simulink model "cbf"  (R2021a)
settings: Solver=FixedStepAuto  StartTime=0.0  StopTime=inf  FixedStep=0.05  RelTol=1e-3
undefined symbols (not defined in the file): Angular, Linear
libraries: robotlib x34
settings Model: Creator=ivory  LastModifiedBy=sprinkle
settings SolverCC: AlgebraicLoopSolver=TrustRegion
settings OptimizationCC: EnhancedBackFolding=on  PassReuseOutputArgsAs=Individual arguments  ZeroExternalMemoryAtStartup=off  ZeroInternalMemoryAtStartup=off  MaxStackSize=64  OptimizeBlockOrder=speed  DifferentSizesBufferReuse=on  OptimizationCustomize=off  EfficientTunableParamExpr=on
settings DebuggingCC: ParameterTunabilityLossMsg=error  SFMachineParentedDataDiag=warning
settings HardwareCC: ProdBitPerPointer=32  ProdBitPerSizeT=32  ProdBitPerPtrDiffT=32  ProdLargestAtomicFloat=None  ProdIntDivRoundTo=Undefined  ProdEndianess=Unspecified  ProdWordSize=32  ProdHWDeviceType=Generic->Unspecified (assume 32-bit Generic)
settings SFSimCC: MATLABDynamicMemAlloc=off  SimTargetLang=C++
settings RTWCC: SystemTargetFile=ert.tlc  HardwareBoard=Robot Operating System (ROS)  TLCOptions="-aInlineSetEventsForThisBaseRateFcn=TLC_FALSE -aSuppressMultiTaskScheduler=TLC_FALSE  -aRateBasedStepFcn=0"  TemplateMakefile=ert_default_tmf  GenerateReport=on  Toolchain=Catkin  IncludeHyperlinkInReport=on  LaunchReport=on  TargetLang=C++  GenerateTraceInfo=on  GenerateTraceReport=on  GenerateTraceReportSl=on  GenerateTraceReportSf=on  GenerateTraceReportEml=on
settings CodeAppCC: ForceParamTrailComments=on  IgnoreCustomStorageClasses=off  OperatorAnnotations=on  SimulinkDataObjDesc=on  SFDataObjDesc=on  InsertBlockDesc=on
settings ERTTargetCC: SupportContinuousTime=on  SupportVariableSizeSignals=on

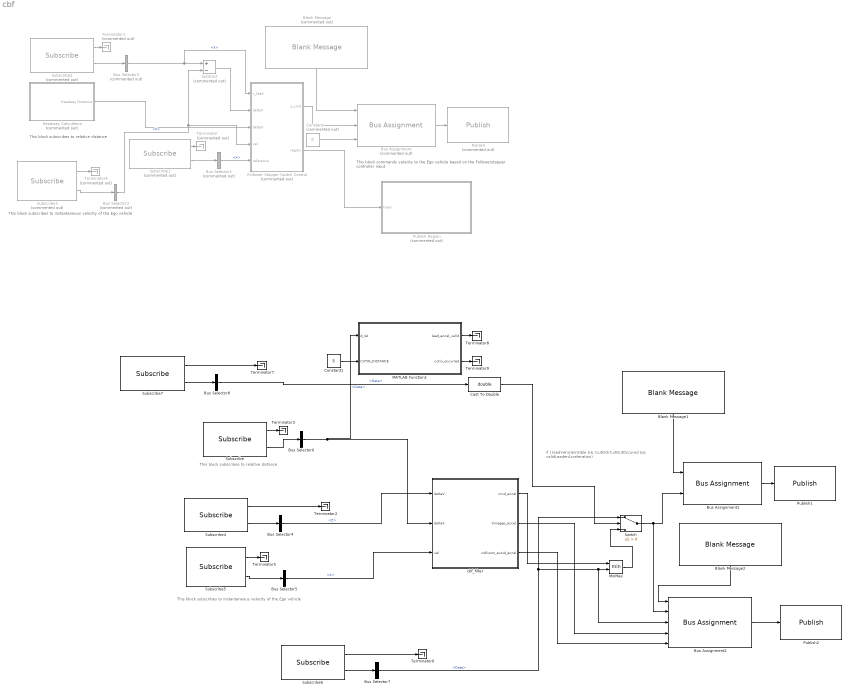
== system cbf ==
  note: if ( leadVehicleVisible && !cutInOrCutOutOccured && validLeaderAcceleration)
  note: This block subscribes to
      | instantaneous velocity of the Ego vehicle
  note: This block subscribes
      | to relative distance
  note: This block commands velocity to the Ego vehicle based
      | on the Followerstopper controller input
  note: This block subscribes
      | to relative distance
  note: This block subscribes to
      | instantaneous velocity of the Ego vehicle
  Blank Message : robotlib/Blank Message  Commented=on  messageClass=Message  entityType=geometry_msgs/Twist  messageType=geometry_msgs/Twist  SampleTime=inf  legacyBusStruct=off
  Blank Message1 : robotlib/Blank Message  messageClass=Message  entityType=std_msgs/Float64  messageType=std_msgs/Float64  SampleTime=inf  legacyBusStruct=off
  Blank Message2 : robotlib/Blank Message  messageClass=Message  entityType=geometry_msgs/Twist  messageType=geometry_msgs/Twist  SampleTime=inf  legacyBusStruct=off
  Bus Assignment : BusAssignment  Commented=on  AssignedSignals=Linear.X,Angular.Z
  Bus Assignment1 : BusAssignment  AssignedSignals=Data
  Bus Assignment2 : BusAssignment  AssignedSignals=Linear.X,Linear.Y,Angular.Y,Angular.Z
  Bus Selector1 : BusSelector  Commented=on  OutputSignals=Linear.X
  Bus Selector2 : BusSelector  Commented=on  OutputSignals=Linear.X
  Bus Selector3 : BusSelector  Commented=on  OutputSignals=Linear.X
  Bus Selector4 : BusSelector  OutputSignals=Linear.Z
  Bus Selector5 : BusSelector  OutputSignals=Linear.X
  Bus Selector6 : BusSelector  OutputSignals=Data
  Bus Selector7 : BusSelector  OutputSignals=Data
  Bus Selector8 : BusSelector  OutputSignals=Data
  Cast To Double : DataTypeConversion  OutDataTypeStr=double
  Constant : Constant  Commented=on  Value=0
  Constant1 : Constant  Value=5
  Follower Stopper Switch Control : Subsystem  Commented=on
  Headway Calculation : Subsystem  Commented=on
  MATLAB Function1 : MATLAB Function  TreatAsAtomicUnit=on
  MinMax : MinMax  Inputs=2
  Publish : robotlib/Publish  Commented=on  topicSource=Specify your own  topic=cmd_vel  messageType=geometry_msgs/Twist  legacyBusStruct=off  messageQueueLength=1
  Publish Region : Subsystem  Commented=on
  Publish1 : robotlib/Publish  topicSource=Specify your own  topic=cmd_accel  messageType=std_msgs/Float64  legacyBusStruct=off  messageQueueLength=1
  Publish2 : robotlib/Publish  topicSource=Specify your own  topic=/cbf/cbf_debug  messageType=geometry_msgs/Twist  legacyBusStruct=off  messageQueueLength=1
  Subscribe : robotlib/Subscribe  topicSource=Specify your own  topic=lead_dist  messageType=std_msgs/Float64  SampleTime=-1  legacyBusStruct=off  messageQueueLength=1
  Subscribe1 : robotlib/Subscribe  Commented=on  topicSource=Specify your own  topic=v_ref  messageType=geometry_msgs/Twist  SampleTime=-1  legacyBusStruct=off  messageQueueLength=1
  Subscribe2 : robotlib/Subscribe  Commented=on  topicSource=Specify your own  topic=leader_vel  messageType=geometry_msgs/Twist  SampleTime=-1  legacyBusStruct=off  messageQueueLength=1
  Subscribe3 : robotlib/Subscribe  Commented=on  topicSource=Specify your own  topic=vel  messageType=geometry_msgs/Twist  SampleTime=-1  legacyBusStruct=off  messageQueueLength=1
  Subscribe4 : robotlib/Subscribe  topicSource=Specify your own  topic=rel_vel  messageType=geometry_msgs/Twist  SampleTime=-1  legacyBusStruct=off  messageQueueLength=1
  Subscribe5 : robotlib/Subscribe  topicSource=Specify your own  topic=vel  messageType=geometry_msgs/Twist  SampleTime=-1  legacyBusStruct=off  messageQueueLength=1
  Subscribe6 : robotlib/Subscribe  topicSource=Specify your own  topic=cmd_accel_pre  messageType=std_msgs/Float64  SampleTime=-1  legacyBusStruct=off  messageQueueLength=1
  Subscribe7 : robotlib/Subscribe  topicSource=Specify your own  topic=/car/hud/mini_car_enable  messageType=std_msgs/Bool  SampleTime=-1  legacyBusStruct=off  messageQueueLength=1
  Subtract : Sum  Commented=on  Inputs=+-
  Switch : Switch  Criteria=u2 > Threshold
  Terminator : Terminator  Commented=on
  Terminator1 : Terminator  Commented=on
  Terminator{2..3,5..9} (7 alike) : Terminator
  Terminator4 : Terminator  Commented=on
  cbf_filter : Subsystem
  wires:
  Bus Assignment/1 -> Publish/1
  Subscribe3/2 -> Bus Selector3/1
  Blank Message/1 -> Bus Assignment/1
  Bus Selector3/1 -> Subtract/2, Follower Stopper Switch Control/4(vel)  "<X>"
  Constant/1 -> Bus Assignment/3
  Subscribe3/1 -> Terminator4/1
  Follower Stopper Switch Control/1(u_cmd) -> Bus Assignment/2
  Headway Calculation/1(Headway Distance) -> Follower Stopper Switch Control/3(deltaX)
  Bus Selector1/1 -> Follower Stopper Switch Control/5(reference)  "<X>"
  Follower Stopper Switch Control/2(region) -> Publish Region/1(Input)
  Subscribe1/1 -> Terminator/1
  Subscribe1/2 -> Bus Selector1/1
  Subscribe2/2 -> Bus Selector2/1
  Bus Selector2/1 -> Follower Stopper Switch Control/1(v_lead), Subtract/1  "<X>"
  Subtract/1 -> Follower Stopper Switch Control/2(deltaV)
  Subscribe2/1 -> Terminator1/1
  Subscribe4/1 -> Terminator2/1
  Bus Selector4/1 -> cbf_filter/1(deltaV)  "<Z>"
  Subscribe5/2 -> Bus Selector5/1
  Subscribe4/2 -> Bus Selector4/1
  Bus Selector5/1 -> cbf_filter/3(vel)  "<X>"
  Bus Assignment1/1 -> Publish1/1
  Blank Message1/1 -> Bus Assignment1/1
  Subscribe5/1 -> Terminator5/1
  Subscribe/1 -> Terminator3/1
  Subscribe/2 -> Bus Selector6/1
  Bus Selector6/1 -> MATLAB Function1/1(d_rel), cbf_filter/2(deltaX)  "<Data>"
  Subscribe6/2 -> Bus Selector7/1
  Bus Selector7/1 -> Switch/1, Bus Assignment2/3, MinMax/2  "<Data>"
  Subscribe6/1 -> Terminator6/1
  Subscribe7/2 -> Bus Selector8/1
  Subscribe7/1 -> Terminator7/1
  Bus Selector8/1 -> Cast To Double/1  "<Data>"
  Constant1/1 -> MATLAB Function1/2(CUTIN_DISTANCE)
  cbf_filter/1(cmd_accel) -> MinMax/1
  MinMax/1 -> Switch/3
  Switch/1 -> Bus Assignment2/2, Bus Assignment1/2
  Blank Message2/1 -> Bus Assignment2/1
  Bus Assignment2/1 -> Publish2/1
  cbf_filter/2(timegap_accel) -> Bus Assignment2/4
  cbf_filter/3(collision_avoid_accel) -> Bus Assignment2/5
  Cast To Double/1 -> Switch/2
  MATLAB Function1/1(lead_accel_valid) -> Terminator8/1
  MATLAB Function1/2(cutin_occurred) -> Terminator9/1

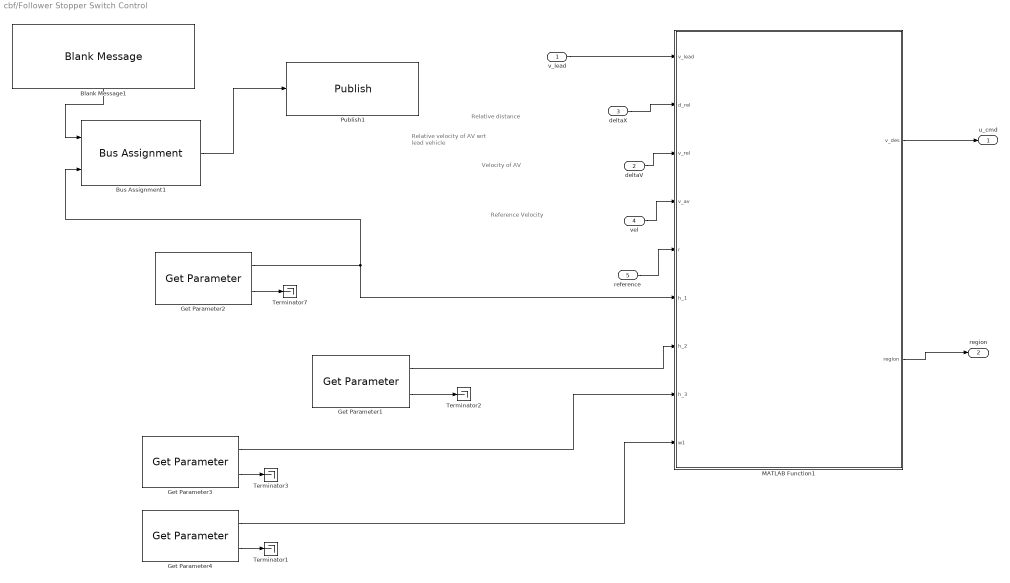
== system cbf/Follower Stopper Switch Control ==
  note: Relative velocity of
      | AV wrt lead vehicle
  note: Velocity of AV
  note: Reference Velocity
  note: Relative distance
  v_lead : Inport
  deltaV : Inport  Port=2
  deltaX : Inport  Port=3
  vel : Inport  Port=4
  reference : Inport  Port=5
  Blank Message1 : robotlib/Blank Message  messageClass=Message  entityType=std_msgs/Float64  messageType=std_msgs/Float64  SampleTime=inf  legacyBusStruct=off
  Bus Assignment1 : BusAssignment  AssignedSignals=Data
  Get Parameter1 : robotlib/Get Parameter  ParameterSource=Specify your own  ParameterName=th2  ParameterType=double  ParameterMaxArrayLength=16  ParameterInitialValue=1.2  SampleTime=-1  ShowErrorCodeOutput=on  ModelName=followerstoppermax  BlockId=ParamGet_followerstoppermax_228
      settings: SourceProductBaseCode=RR
  Get Parameter2 : robotlib/Get Parameter  ParameterSource=Specify your own  ParameterName=th1  ParameterType=double  ParameterMaxArrayLength=16  ParameterInitialValue=0.4  SampleTime=-1  ShowErrorCodeOutput=on  ModelName=followerstoppermax  BlockId=ParamGet_followerstoppermax_226
      settings: SourceProductBaseCode=RR
  Get Parameter3 : robotlib/Get Parameter  ParameterSource=Specify your own  ParameterName=th3  ParameterType=double  ParameterMaxArrayLength=16  ParameterInitialValue=1.8  SampleTime=-1  ShowErrorCodeOutput=on  ModelName=followerstoppermax  BlockId=ParamGet_followerstoppermax_230
      settings: SourceProductBaseCode=RR
  Get Parameter4 : robotlib/Get Parameter  ParameterSource=Specify your own  ParameterName=w1  ParameterType=double  ParameterMaxArrayLength=16  ParameterInitialValue=4.5  SampleTime=-1  ShowErrorCodeOutput=on  ModelName=followerstoppermax  BlockId=ParamGet_followerstoppermax_235
      settings: SourceProductBaseCode=RR
  MATLAB Function1 : MATLAB Function  TreatAsAtomicUnit=on
  Publish1 : robotlib/Publish  topicSource=Specify your own  topic=timheadway1  messageType=std_msgs/Float64  legacyBusStruct=off  messageQueueLength=1
  Terminator{1..3,7} (4 alike) : Terminator
  u_cmd : Outport
  region : Outport  Port=2
  wires:
  deltaX/1 -> MATLAB Function1/2(d_rel)
  deltaV/1 -> MATLAB Function1/3(v_rel)
  vel/1 -> MATLAB Function1/4(v_av)
  v_lead/1 -> MATLAB Function1/1(v_lead)
  reference/1 -> MATLAB Function1/5(r)
  MATLAB Function1/1(v_des) -> u_cmd/1
  MATLAB Function1/2(region) -> region/1
  Get Parameter3/1 -> MATLAB Function1/8(h_3)
  Get Parameter1/2 -> Terminator2/1
  Get Parameter1/1 -> MATLAB Function1/7(h_2)
  Get Parameter3/2 -> Terminator3/1
  Get Parameter2/2 -> Terminator7/1
  Blank Message1/1 -> Bus Assignment1/1
  Bus Assignment1/1 -> Publish1/1
  Get Parameter2/1 -> Bus Assignment1/2, MATLAB Function1/6(h_1)
  Get Parameter4/2 -> Terminator1/1
  Get Parameter4/1 -> MATLAB Function1/9(w1)

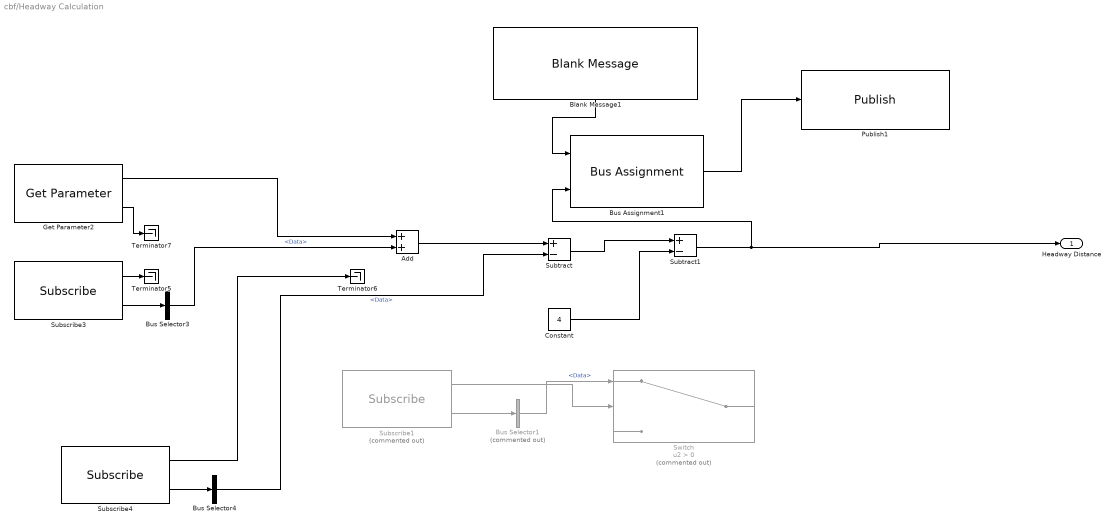
== system cbf/Headway Calculation ==
  Add : Sum
  Blank Message1 : robotlib/Blank Message  messageClass=Message  entityType=std_msgs/Float64  messageType=std_msgs/Float64  SampleTime=inf  legacyBusStruct=off
  Bus Assignment1 : BusAssignment  AssignedSignals=Data
  Bus Selector1 : BusSelector  Commented=on  OutputSignals=Data
  Bus Selector3 : BusSelector  OutputSignals=Data
  Bus Selector4 : BusSelector  OutputSignals=Data
  Constant : Constant  Value=4
  Get Parameter2 : robotlib/Get Parameter  ParameterSource=Specify your own  ParameterName=init_gap  ParameterType=double  ParameterMaxArrayLength=16  ParameterInitialValue=30.0  SampleTime=-1  ShowErrorCodeOutput=on  ModelName=fs_th  BlockId=ParamGet_fs_th_177
      settings: SourceProductBaseCode=RR
  Publish1 : robotlib/Publish  topicSource=Specify your own  topic=headway_est  messageType=std_msgs/Float64  legacyBusStruct=off  messageQueueLength=1
  Subscribe1 : robotlib/Subscribe  Commented=on  topicSource=Specify your own  topic=headway  messageType=std_msgs/Float64  SampleTime=-1  legacyBusStruct=off  messageQueueLength=1
  Subscribe3 : robotlib/Subscribe  topicSource=Specify your own  topic=leader_dist_x  messageType=std_msgs/Float64  SampleTime=-1  legacyBusStruct=off  messageQueueLength=1
  Subscribe4 : robotlib/Subscribe  topicSource=Specify your own  topic=dist_x  messageType=std_msgs/Float64  SampleTime=-1  legacyBusStruct=off  messageQueueLength=1
  Subtract : Sum  Inputs=+-
  Subtract1 : Sum  Inputs=+-
  Switch : Switch  Commented=on  Criteria=u2 > Threshold
  Terminator5 : Terminator
  Terminator6 : Terminator
  Terminator7 : Terminator
  Headway Distance : Outport
  wires:
  Bus Selector3/1 -> Add/2  "<Data>"
  Subscribe1/2 -> Bus Selector1/1
  Subscribe3/2 -> Bus Selector3/1
  Subscribe4/1 -> Terminator6/1
  Bus Selector1/1 -> Switch/1  "<Data>"
  Subscribe1/1 -> Switch/2
  Bus Selector4/1 -> Subtract/2  "<Data>"
  Get Parameter2/2 -> Terminator7/1
  Subscribe4/2 -> Bus Selector4/1
  Get Parameter2/1 -> Add/1
  Subscribe3/1 -> Terminator5/1
  Add/1 -> Subtract/1
  Subtract/1 -> Subtract1/1
  Blank Message1/1 -> Bus Assignment1/1
  Bus Assignment1/1 -> Publish1/1
  Subtract1/1 -> Bus Assignment1/2, Headway Distance/1
  Constant/1 -> Subtract1/2

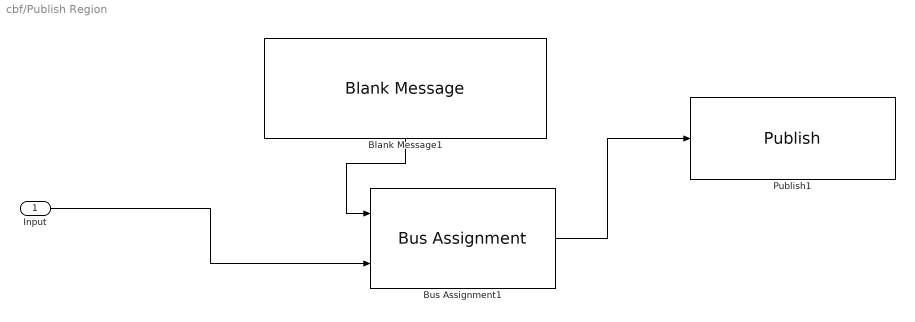
== system cbf/Publish Region ==
  Input : Inport
  Blank Message1 : robotlib/Blank Message  messageClass=Message  entityType=std_msgs/UInt8  messageType=std_msgs/UInt8  SampleTime=inf  legacyBusStruct=off
  Bus Assignment1 : BusAssignment  AssignedSignals=Data
  Publish1 : robotlib/Publish  topicSource=Specify your own  topic=region  messageType=std_msgs/UInt8  legacyBusStruct=off  messageQueueLength=1
  wires:
  Input/1 -> Bus Assignment1/2
  Blank Message1/1 -> Bus Assignment1/1
  Bus Assignment1/1 -> Publish1/1

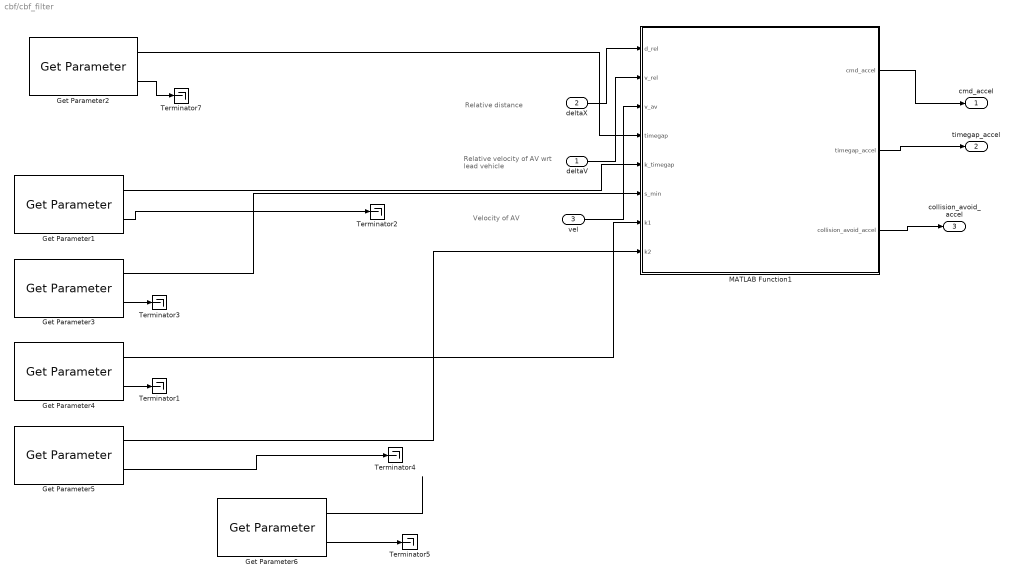
== system cbf/cbf_filter ==
  note: Velocity of AV
  note: Relative velocity of
      | AV wrt lead vehicle
  note: Relative distance
  deltaV : Inport
  deltaX : Inport  Port=2
  vel : Inport  Port=3
  Get Parameter1 : robotlib/Get Parameter  ParameterSource=Specify your own  ParameterName=k_timegap  ParameterType=double  ParameterMaxArrayLength=16  ParameterInitialValue=0.1  SampleTime=-1  ShowErrorCodeOutput=on  ModelName=cbf  BlockId=ParamGet_cbf_447
      settings: SourceProductBaseCode=RR
  Get Parameter2 : robotlib/Get Parameter  ParameterSource=Specify your own  ParameterName=timegap  ParameterType=double  ParameterMaxArrayLength=16  ParameterInitialValue=2.0  SampleTime=-1  ShowErrorCodeOutput=on  ModelName=cbf  BlockId=ParamGet_cbf_448
      settings: SourceProductBaseCode=RR
  Get Parameter3 : robotlib/Get Parameter  ParameterSource=Specify your own  ParameterName=s_min  ParameterType=double  ParameterMaxArrayLength=16  ParameterInitialValue=15.0  SampleTime=-1  ShowErrorCodeOutput=on  ModelName=cbf  BlockId=ParamGet_cbf_449
      settings: SourceProductBaseCode=RR
  Get Parameter4 : robotlib/Get Parameter  ParameterSource=Specify your own  ParameterName=k1  ParameterType=double  ParameterMaxArrayLength=16  ParameterInitialValue=0.5  SampleTime=-1  ShowErrorCodeOutput=on  ModelName=cbf  BlockId=ParamGet_cbf_450
      settings: SourceProductBaseCode=RR
  Get Parameter5 : robotlib/Get Parameter  ParameterSource=Specify your own  ParameterName=k2  ParameterType=double  ParameterMaxArrayLength=16  ParameterInitialValue=0.5  SampleTime=-1  ShowErrorCodeOutput=on  ModelName=cbf  BlockId=ParamGet_cbf_463
      settings: SourceProductBaseCode=RR
  Get Parameter6 : robotlib/Get Parameter  ParameterSource=Specify your own  ParameterName=w3  ParameterType=double  ParameterMaxArrayLength=16  ParameterInitialValue=6.0  SampleTime=-1  ShowErrorCodeOutput=on  ModelName=cbf  BlockId=ParamGet_cbf_465
      settings: SourceProductBaseCode=RR
  MATLAB Function1 : MATLAB Function  TreatAsAtomicUnit=on
  Terminator{1..5,7} (6 alike) : Terminator
  cmd_accel : Outport
  timegap_accel : Outport  Port=2
  collision_avoid_accel : Outport  Port=3
  wires:
  Get Parameter4/1 -> MATLAB Function1/7(k1)
  Get Parameter4/2 -> Terminator1/1
  Get Parameter2/1 -> MATLAB Function1/4(timegap)
  Get Parameter2/2 -> Terminator7/1
  Get Parameter3/2 -> Terminator3/1
  Get Parameter1/1 -> MATLAB Function1/5(k_timegap)
  Get Parameter1/2 -> Terminator2/1
  Get Parameter3/1 -> MATLAB Function1/6(s_min)
  MATLAB Function1/2(timegap_accel) -> timegap_accel/1
  MATLAB Function1/1(cmd_accel) -> cmd_accel/1
  vel/1 -> MATLAB Function1/3(v_av)
  deltaV/1 -> MATLAB Function1/2(v_rel)
  deltaX/1 -> MATLAB Function1/1(d_rel)
  Get Parameter5/2 -> Terminator4/1
  Get Parameter5/1 -> MATLAB Function1/8(k2)
  Get Parameter6/1 -> ?
  Get Parameter6/2 -> Terminator5/1
  MATLAB Function1/3(collision_avoid_accel) -> collision_avoid_accel/1

== matlab function cbf/Follower Stopper Switch Control/MATLAB Function1 ==
  data: v_lead input; v_des output; d_rel input; v_rel input; v_av input; r input; region output; h_1 input; h_2 input; h_3 input; w1 input
function [v_des, region]= fcn(v_lead, d_rel,v_rel,v_av, r, h_1, h_2, h_3, w1)
%#codegen
% Safety controller, based on quadratic bands.
% Input: r = desired velocity (from other models)
%          d_rel = estimate of gap to vehicle ahead
%          v_rel = estimate of time derivative of dx (= velocity difference)
%         v_AV = velocity of AV
%      dx_min = minimum distance
% dx_activate = distance below which controller does something
%       decel = vector of three deceleration values for parabolas
% Out:  u_cmd = actual velocity commanded (always u_cmd<=U)
%
% Controller-specific parameters

    w = zeros(3,1);
    alpha = zeros(3,1);
    w(1) = w1;
    alpha(1) = 1.5;
    w(3) = 6.0;
    alpha(3) = 0.5;
    w(2) = (w(1)+w(3))/2;
    alpha(2) = (alpha(1)+alpha(3))/2;
    if(nargin<4)
        r = 30;
    end
    
    %v_rel_star = min(v_rel,0)
    v_rel_star = v_rel;
    v_rel_star(v_rel >= 0) = 0;
    
%     h_1 = 0.4;
%     h_2 = 1.2;
%     h_3 = 1.8;
    
    x1 = (0.5*v_rel_star.^2)/alpha(1) + max(h_1*v_av,w(1));
    x2 = (0.5*v_rel_star.^2)/alpha(2) + max(h_2*v_av,w(2));
    x3 = (0.5*v_rel_star.^2)/alpha(3) + max(h_3*v_av,w(3));
    
%     v_lead = v_av+v_rel;
    
    
    %v = min([max([v_lead,0]),r]);
    v = v_lead;
    v(v_lead<0) = 0;
    
    v(v_lead>r) = r;
  
    v_des = zeros(size(d_rel)); 
    %safe region
    v_des(d_rel>x3) = r;  
    %adaptation region 2
    temp_v_des = v+(r-v).*(d_rel-x2)./(x3-x2);
    v_des(d_rel>x2 & d_rel<=x3) = temp_v_des(d_rel>x2 & d_rel<=x3);   
    %adaptation region 1
    temp_v_des = v.*(d_rel-x1)./(x2-x1);
    v_des(d_rel>x1 & d_rel<=x2) = temp_v_des(d_rel>x1 & d_rel<=x2); 
    
    if d_rel>x3
        region = uint8(0);
    elseif d_rel>x2 && d_rel<=x3
        region = uint8(1);
    elseif d_rel>x1 && d_rel<=x2
        region = uint8(2);
    else
        region = uint8(3);
    end

== matlab function cbf/cbf_filter/MATLAB Function1 ==
  data: cmd_accel output; d_rel input; v_rel input; v_av input; timegap input; timegap_accel output; collision_avoid_accel output; k_timegap input; s_min input; k1 input; k2 input
function [cmd_accel, timegap_accel, collision_avoid_accel]= fcn(d_rel,v_rel,v_av, timegap,k_timegap,s_min,k1,k2)
%#codegen

% from the timegap filter function
% maybe make this gain a parameter later
% k = 0.1;
k = k_timegap;
%t_min = 2.0;
t_min = timegap;
timegap_accel = (1/t_min)*v_rel + (k/t_min)*(d_rel - t_min*v_av);

% from collision-avoid filter function
% a potential parameter - read into the fcn now
% s_min = 15.0;
% a potential parameter - read into the fcn now
% k1 = 0.5;
% a potential parameter - read into the fcn now
% k2 = 0.5;
%a_max = a_l + (k1+k2)*(delta_v) + (k1*k2)*(s-s_min);
% simplification TODO this is maybe dangerous so need to confirm
a_l = 0;
collision_avoid_accel = a_l + (k1+k2)*(v_rel) + (k1*k2)*(d_rel-s_min);

% now put these together
% 	 tg_accel = time_gap_filter(v,s,delta_v)
% 	 ca_accel = collision_avoid_filter(s,delta_v,a_l)
% 	 return min([tg_accel,ca_accel])
% TODO make max/min acceleration parameters.
cmd_accel = min(1.5,max(-3.0,min(timegap_accel,collision_avoid_accel)));

== matlab function cbf/MATLAB Function1 ==
  data: lead_accel_valid output; d_rel input; CUTIN_DISTANCE input; cutin_occurred output
function [lead_accel_valid, cutin_occurred]= fcn(d_rel,CUTIN_DISTANCE)
%#codegen

persistent relative_distance_prev;
if isempty(relative_distance_prev)
    relative_distance_prev=d_rel;
end

cutin_occurred = 1;
lead_accel_valid=1;

if( abs( relative_distance_prev - d_rel ) > CUTIN_DISTANCE )
    cutin_occurred = 1;
else
    cutin_occurred = 0;
end

relative_distance_prev = d_rel;
